simulink model "washout"  (R2018b)
settings: Solver=VariableStepAuto  StartTime=0.0  StopTime=30  RelTol=1e-3
settings Model: Creator=15705  LastModifiedBy=15705

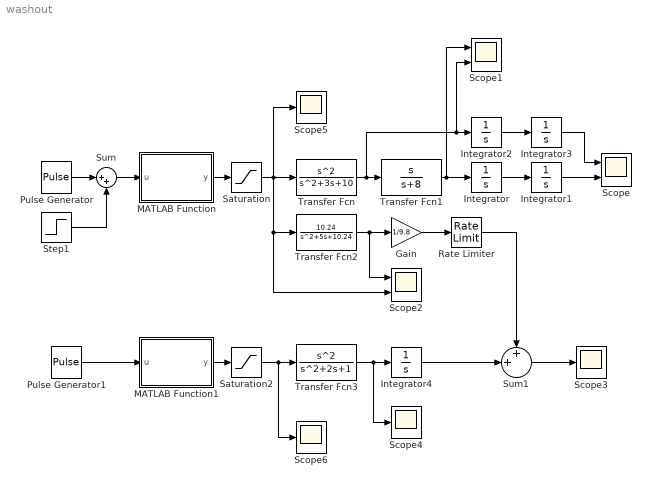
== system washout ==
  Gain : Gain  Gain=1/9.8
  Integrator{,1..4} (5 alike) : Integrator
  MATLAB Function : MATLAB Function  TreatAsAtomicUnit=on
  MATLAB Function1 : MATLAB Function  TreatAsAtomicUnit=on
  Pulse Generator : DiscretePulseGenerator  PulseType=Time based  Period=100  PulseWidth=5  PhaseDelay=3
  Pulse Generator1 : DiscretePulseGenerator  PulseType=Time based  Period=100  PulseWidth=5  PhaseDelay=3
  Rate Limiter : RateLimiter  RisingSlewLimit=0.052  FallingSlewLimit=-0.052  SampleTimeMode=inherited
  Saturation : Saturate  UpperLimit=2.5  LowerLimit=-2.5
  Saturation2 : Saturate  UpperLimit=2.5  LowerLimit=-2.5
  Scope : Scope  NumInputPorts=2
  Scope1 : Scope  NumInputPorts=2
  Scope2 : Scope  NumInputPorts=2
  Scope{3..6} (4 alike) : Scope
  Step1 : Step  Time=0  After=0  SampleTime=0
  Sum : Sum  Inputs=|++
  Sum1 : Sum  Inputs=++|
  Transfer Fcn : TransferFcn  Numerator=[1 0 0]  Denominator=[1 3 10]
  Transfer Fcn1 : TransferFcn  Numerator=[1 0]  Denominator=[1 8]
  Transfer Fcn2 : TransferFcn  Numerator=[10.24]  Denominator=[1 5 10.24]
  Transfer Fcn3 : TransferFcn  Numerator=[1 0 0]
  wires:
  Pulse Generator/1 -> Sum/1
  Sum/1 -> MATLAB Function/1(u)
  MATLAB Function/1(y) -> Saturation/1
  Transfer Fcn/1 -> Integrator2/1, Scope1/2, Transfer Fcn1/1
  Transfer Fcn1/1 -> Integrator/1, Scope1/1
  Saturation/1 -> Scope5/1, Scope2/2, Transfer Fcn2/1, Transfer Fcn/1
  Step1/1 -> Sum/2
  Integrator1/1 -> Scope/2
  Integrator3/1 -> Scope/1
  Integrator/1 -> Integrator1/1
  Integrator2/1 -> Integrator3/1
  MATLAB Function1/1(y) -> Saturation2/1
  Transfer Fcn2/1 -> Scope2/1, Gain/1
  Gain/1 -> Rate Limiter/1
  Saturation2/1 -> Scope6/1, Transfer Fcn3/1
  Transfer Fcn3/1 -> Scope4/1, Integrator4/1
  Integrator4/1 -> Sum1/2
  Sum1/1 -> Scope3/1
  Pulse Generator1/1 -> MATLAB Function1/1(u)
  Rate Limiter/1 -> Sum1/1

== matlab function washout/MATLAB Function1 ==
  data: u input; y output
function y = fcn(u)

y=-0.001*u^3-0.03*u^2+u;

== matlab function washout/MATLAB Function ==
  data: u input; y output
function y = fcn(u)

y=-0.001*u^3-0.03*u^2+u;
